simulink model "TestSerial"  (R2012b)
settings: Solver=ode45  StartTime=0.0  StopTime=inf  RelTol=1e-3
undefined symbols (not defined in the file or in its folder): CR, serial
libraries: instrumentlib x2, realtime_pacer_lib x1
settings Model: Creator=Thomas  LastModifiedBy=Thomas

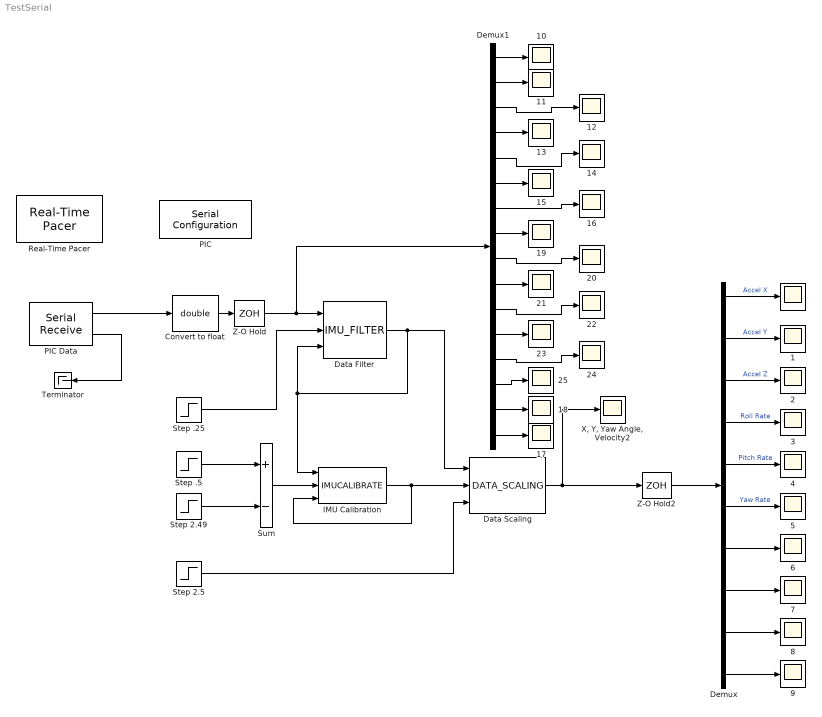
== system TestSerial ==
   {,1..25} (26 alike) : Scope
      " " settings: TimeRange=10  YMin=-12.5  YMax=45
      " 1" settings: TimeRange=10  YMin=-12.5  YMax=45  SaveName=ScopeData2
      " 10" settings: TimeRange=10  YMin=1  YMax=1  SaveName=ScopeData11
      " 11" settings: TimeRange=10  YMin=0.95  YMax=1.05  SaveName=ScopeData12
      " 12" settings: TimeRange=10  YMin=1  YMax=1  SaveName=ScopeData13
      " 13" settings: TimeRange=10  YMin=0.95  YMax=1.05  SaveName=ScopeData14
      " 14" settings: TimeRange=10  YMin=3  YMax=3  SaveName=ScopeData15
      " 15" settings: TimeRange=10  YMin=0.95  YMax=1.05  SaveName=ScopeData16
      " 16" settings: TimeRange=10  YMin=2  YMax=2  SaveName=ScopeData17
      " 17" settings: TimeRange=10  YMin=0.95  YMax=1.05  SaveName=ScopeData18
      " 18" settings: TimeRange=10  YMin=0  YMax=32.5  SaveName=ScopeData19
      " 19" settings: TimeRange=10  YMin=1.9  YMax=2.1  SaveName=ScopeData20
      " 2" settings: TimeRange=10  YMin=-12.5  YMax=45  SaveName=ScopeData3
      " 20" settings: TimeRange=10  YMin=1.9  YMax=2.1  SaveName=ScopeData21
      " 21" settings: TimeRange=10  YMin=1.9  YMax=2.1  SaveName=ScopeData22
      " 22" settings: TimeRange=10  YMin=1.9  YMax=2.1  SaveName=ScopeData23
      " 23" settings: TimeRange=10  YMin=1.9  YMax=2.1  SaveName=ScopeData24
      " 24" settings: TimeRange=10  YMin=1.9  YMax=2.1  SaveName=ScopeData25
      " 25" settings: TimeRange=10  YMin=1.9  YMax=2.1  SaveName=ScopeData26
      " 3" settings: TimeRange=10  YMin=-12.5  YMax=45  SaveName=ScopeData4
      " 4" settings: TimeRange=10  YMin=-12.5  YMax=45  SaveName=ScopeData5
      " 5" settings: TimeRange=10  YMin=-12.5  YMax=45  SaveName=ScopeData6
      " 6" settings: TimeRange=10  YMin=-12.5  YMax=45  SaveName=ScopeData7
      " 7" settings: TimeRange=10  YMin=-12.5  YMax=45  SaveName=ScopeData8
      " 8" settings: TimeRange=10  YMin=-12.5  YMax=45  SaveName=ScopeData9
      " 9" settings: TimeRange=10  YMin=-12.5  YMax=45  SaveName=ScopeData10
  Convert to float : DataTypeConversion  OutDataTypeStr=double  SaturateOnIntegerOverflow=on  RndMeth=Zero
  Data Filter : M-S-Function  FunctionName=IMU_FILTER  Parameters=3
  "Data Scaling " : M-S-Function  FunctionName=DATA_SCALING  Parameters=3
  Demux : Demux  Outputs=10
  Demux1 : Demux  Outputs=16
  IMU Calibration : M-S-Function  FunctionName=IMUCALIBRATE  Parameters=3
  PIC : instrumentlib/Serial Configuration  Priority=-200000  ComPortMenu=COM11  ComPort=COM11  ObjConstructor=serial('COM11');  BaudRate=9600  DataBits=8  Parity=none  StopBits=1  FlowControl=none  Timeout=10  ByteOrder=LittleEndian
  PIC Data : instrumentlib/Serial Receive  ComPortMenu=COM11  ComPort=COM11  ObjConstructor=serial('COM11');  Terminator=CR ('\r')  DataSize="[1  16]"  DataType=uint8  EnableBlockingMode=off  ActionDataUnavailable=Output last received value  CustomValue=0  SampleTime=.05
  Real-Time Pacer : realtime_pacer_lib/Real-Time Pacer  simTimePerRealTime=1
  Step .25 : Step  Time=.25  SampleTime=0
  Step .5 : Step  Time=.5  SampleTime=0
  Step 2.49 : Step  Time=2.49  SampleTime=0
  Step 2.5 : Step  Time=2.5  SampleTime=0
  Sum : Sum  Inputs=+-
  Terminator : Terminator
  "X, Y, Yaw Angle, Velocity2" : Scope
      settings: TimeRange=10  YMin=-12.5  YMax=45
  Z-O Hold : ZeroOrderHold  SampleTime=0.05
  Z-O Hold2 : ZeroOrderHold  SampleTime=0.05
  wires:
  PIC Data/2 -> Terminator/1
  Convert to float/1 -> Z-O Hold/1
  Data Filter/1 -> "Data Scaling "/1, IMU Calibration/1, Data Filter/3
  IMU Calibration/1 -> IMU Calibration/3, "Data Scaling "/2
  Step .5/1 -> Sum/1
  Step 2.49/1 -> Sum/2
  Z-O Hold/1 -> Demux1/1, Data Filter/1
  Step .25/1 -> Data Filter/2
  Sum/1 -> IMU Calibration/2
  Step 2.5/1 -> "Data Scaling "/3
  "Data Scaling "/1 -> Z-O Hold2/1, "X, Y, Yaw Angle, Velocity2"/1
  PIC Data/1 -> Convert to float/1
  Demux/2 -> " 1"/1  "Accel Y"
  Demux/5 -> " 4"/1  "Pitch Rate"
  Z-O Hold2/1 -> Demux/1
  Demux/1 -> " "/1  "Accel X"
  Demux/3 -> " 2"/1  "Accel Z"
  Demux/4 -> " 3"/1  "Roll Rate"
  Demux/6 -> " 5"/1  "Yaw Rate"
  Demux/7 -> " 6"/1
  Demux/8 -> " 7"/1
  Demux/9 -> " 8"/1
  Demux/10 -> " 9"/1
  Demux1/1 -> " 10"/1
  Demux1/2 -> " 11"/1
  Demux1/3 -> " 12"/1
  Demux1/4 -> " 13"/1
  Demux1/5 -> " 14"/1
  Demux1/6 -> " 15"/1
  Demux1/7 -> " 16"/1
  Demux1/16 -> " 17"/1
  Demux1/15 -> " 18"/1
  Demux1/8 -> " 19"/1
  Demux1/9 -> " 20"/1
  Demux1/10 -> " 21"/1
  Demux1/11 -> " 22"/1
  Demux1/12 -> " 23"/1
  Demux1/13 -> " 24"/1
  Demux1/14 -> " 25"/1
